simulink model "GA_tunning"  (R2019a)
settings: Solver=VariableStepAuto  StartTime=0.0  StopTime=200  RelTol=1e-3
libraries: fuzblock x1
settings Model: Creator=ADHM  LastModifiedBy=ADHM
settings DataIOCC: ReturnWorkspaceOutputs=off

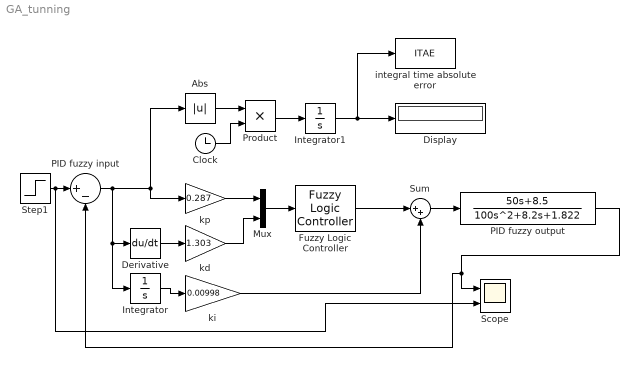
== system GA_tunning ==
  Abs : Abs
  Clock : Clock
  Derivative : Derivative
  Display : Display
  Fuzzy Logic Controller : fuzblock/Fuzzy Logic  Controller  FIS='PID_like_fuzzy_sugeno.fis'  OutputSampleNumber=101  DataType=double  FuzzifiedInputs=off  RuleFiringStrengths=off  RuleOutputs=off  AggregatedOutputs=off  SimulateUsing=Interpreted execution  OutOfRangeInputValueMessage=warning  NoRuleFiredMessage=warning  EmptyOutputFuzzySetMessage=warning
  Integrator : Integrator
  Integrator1 : Integrator
  Mux : Mux  Inputs=2
  "PID fuzzy input " : Sum  Inputs=|+-
  PID fuzzy output : TransferFcn  Numerator=[50 8.5]  Denominator=[100 8.2 1.822]
  Product : Product
  Scope : Scope  NumInputPorts=2
  Step1 : Step  After=30  SampleTime=0
  Sum : Sum  Inputs=|++
  integral time absolute error : ToWorkspace  VariableName=ITAE  SampleTime=-1
  kd : Gain  Gain=1.303
  ki : Gain  Gain=0.00998
  kp : Gain  Gain=0.287
  wires:
  Integrator1/1 -> integral time absolute error/1, Display/1
  Step1/1 -> Scope/2, "PID fuzzy input "/1
  ki/1 -> Sum/2
  Derivative/1 -> kd/1
  PID fuzzy output/1 -> Scope/1, "PID fuzzy input "/2
  kd/1 -> Mux/2
  "PID fuzzy input "/1 -> Abs/1, kp/1, Integrator/1, Derivative/1
  Integrator/1 -> ki/1
  kp/1 -> Mux/1
  Product/1 -> Integrator1/1
  Sum/1 -> PID fuzzy output/1
  Abs/1 -> Product/1
  Clock/1 -> Product/2
  Mux/1 -> Fuzzy Logic Controller/1
  Fuzzy Logic Controller/1 -> Sum/1
